simulink model "task1"  (R2025a)
settings: Solver=VariableStepAuto  StartTime=0.0  StopTime=10.0  RelTol=1e-3
undefined symbols (not defined in the file): Kob, Ti1, Ti2, Ti3, Tint, Tmu
settings Model: Creator=zuimio  LastModifiedBy=zuimio

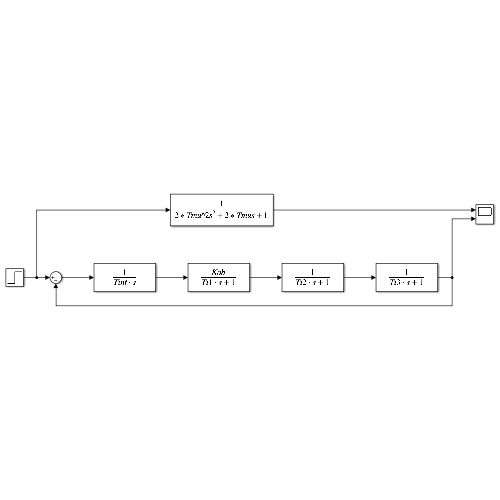
[thumbnail: Simulink's stored preview of the top-level diagram]
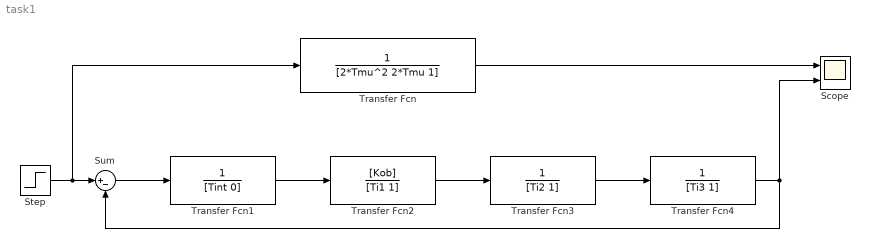
== system task1 ==
  Scope : Scope  NumInputPorts=2
  Step : Step  SampleTime=0
  Sum : Sum  Inputs=|+-
  Transfer Fcn : TransferFcn  Denominator=[2*Tmu^2 2*Tmu 1]
  Transfer Fcn1 : TransferFcn  Denominator=[Tint 0]
  Transfer Fcn2 : TransferFcn  Numerator=[Kob]  Denominator=[Ti1 1]
  Transfer Fcn3 : TransferFcn  Numerator=1  Denominator=[Ti2 1]
  Transfer Fcn4 : TransferFcn  Numerator=1  Denominator=[Ti3 1]
  wires:
  Transfer Fcn1/1 -> Transfer Fcn2/1
  Transfer Fcn2/1 -> Transfer Fcn3/1
  Transfer Fcn3/1 -> Transfer Fcn4/1
  Sum/1 -> Transfer Fcn1/1
  Transfer Fcn4/1 -> Sum/2, Scope/2
  Step/1 -> Transfer Fcn/1, Sum/1
  Transfer Fcn/1 -> Scope/1
